simulink model "PV"  (Simulink 8.3)
settings: Solver=ode45  StartTime=0.0  StopTime=0.7  RelTol=1e-3
undefined symbols (not defined in the file or in its folder): ln
libraries: simulink x3, powerlib x1
settings Model: Creator=Birdman  LastModifiedBy=jt  SimulationMode=accelerator
settings OptimizationCC: InitFltsAndDblsToZero=on  EfficientMapNaN2IntZero=off
settings DebuggingCC: SaveWithParameterizedLinksMsg=none  SignalResolutionControl=TryResolveAllWithWarning  FcnCallInpInsideContextMsg=UseLocalSettings  StateNameClashWarn=none
settings HardwareCC: TargetIntDivRoundTo=Zero  TargetEndianess=LittleEndian  TargetHWDeviceType=MATLAB Host  ProdEqTarget=off
settings CodeAppCC: MaxIdLength=128
settings ConfigurationSet: Description=SimMechanics 2G

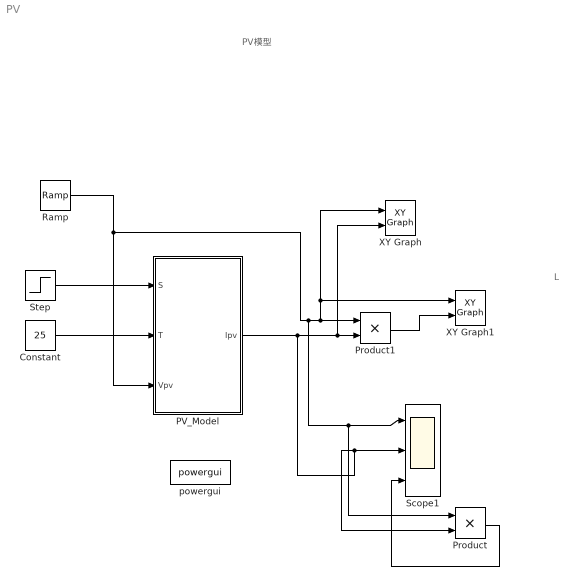
== system PV ==
  note: PV模型
  note: L
  Constant : Constant  Value=25
  PV_Model : Subsystem  mask{Vm=288, Im=13.88, Voc=354, Isc=14.88, Sref=1000, Tref=25, a=0.0025, b=0.0028, Rs=0.5}
      mask prompts: a "a(A/C)"; b "b(V/C)"
      mask Display: disp('PV_array')
  Product : Product
  Product1 : Product
  Ramp : simulink/Sources/Ramp  slope=800  start=0  X0=0
  Scope1 : Scope  NumInputPorts=3
      settings: YMin=255.75~14.58~3737.5  YMax=258.5~14.6125~3770
  Step : Step  Time=0.3  Before=1000  After=1000  SampleTime=0
  XY Graph : simulink/Sinks/XY Graph  xmin=0  xmax=400  ymin=0  ymax=20  st=-1
  XY Graph1 : simulink/Sinks/XY Graph  xmin=0  xmax=400  ymin=0  ymax=4100  st=-1
  powergui : powerlib/powergui  SimulationMode=Discrete  SolverType=Tustin  SampleTime=1e-6  frequency=60  SPID=off  DisableSnubberDevices=off  DisableRonSwitches=off  DisableVfSwitches=off  SwTol=0  Interpol=off  DisplayEquations=off  Ts=0  methode=off  frequencyindice=0  Pbase=100e6  ErrMax=1e-4  Iterations=50  UnitsV=kV  UnitsW=MW  FunctionMessages=off  echomessages=off  HookPort=off  EnableUseOfTLC=off  x0status=blocks  RestoreLinks=warning  ResistiveCurrentMeasurement=off  Frange=[0:2:500]  Ylog=off  Xlog=on  ShowGrid=off  save=off  variable=ZData  structure=io  ZoomFFT=off  StartTime=0.0  cycles=3  DisplayStyle=1  fundamental=50  FreqAxis=on  MaxFrequency=2500  frequencyindicesteady=1  RmsSteady=1  display=off
  wires:
  Step/1 -> PV_Model/1(S)
  Constant/1 -> PV_Model/2(T)
  Ramp/1 -> Product/1, Scope1/1, XY Graph/1, XY Graph1/1, Product1/1, PV_Model/3(Vpv)
  PV_Model/1(Ipv) -> Product/2, Scope1/2, XY Graph/2, Product1/2
  Product/1 -> Scope1/3
  Product1/1 -> XY Graph1/2

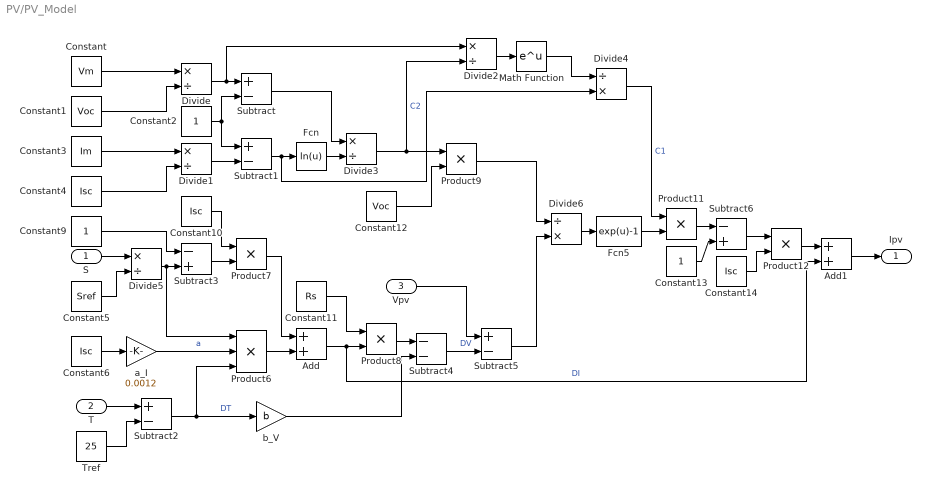
== system PV/PV_Model ==
  S : Inport
  T : Inport  Port=2
  Vpv : Inport  Port=3
  Add : Sum
  Add1 : Sum
  Constant : Constant  Value=Vm
  Constant1 : Constant  Value=Voc
  Constant{4,6,10,14} (4 alike) : Constant  Value=Isc
  Constant11 : Constant  Value=Rs
  Constant12 : Constant  Value=Voc
  Constant13 : Constant
  Constant2 : Constant
  Constant3 : Constant  Value=Im
  Constant5 : Constant  Value=Sref
  Constant9 : Constant
  Divide{,1..3,5} (5 alike) : Product  Inputs=*/
  Divide4 : Product  Inputs=/*
  Divide6 : Product  Inputs=/*
  Fcn : Fcn  Expr=ln(u)
  Fcn5 : Fcn  Expr=exp(u)-1
  Math Function : Math  SaturateOnIntegerOverflow=on
  Product{7..9,11..12} (5 alike) : Product  RndMeth=Zero
  Product6 : Product  Inputs=3  RndMeth=Zero
  Subtract{,1..2,5} (4 alike) : Sum  Inputs=+-
  Subtract3 : Sum  Inputs=-+
  Subtract4 : Sum  Inputs=--
  Subtract6 : Sum  Inputs=-+
  Tref : Constant  Value=25
  a_I : Gain  Gain=0.0012
  b_V : Gain  Gain=b
  Ipv : Outport
  wires:
  Constant1/1 -> Divide/2
  Constant/1 -> Divide/1
  Divide/1 -> Subtract/1, Divide2/1
  Constant2/1 -> Subtract/2, Subtract1/1
  Constant4/1 -> Divide1/2
  Constant3/1 -> Divide1/1
  Divide1/1 -> Subtract1/2
  Subtract1/1 -> Divide4/2, Fcn/1
  Subtract/1 -> Divide3/1
  Divide3/1 -> Product9/1, Divide2/2  "C2"
  Divide2/1 -> Math Function/1
  Math Function/1 -> Divide4/1
  Divide4/1 -> Product11/1  "C1"
  T/1 -> Subtract2/1
  Tref/1 -> Subtract2/2
  Subtract2/1 -> Product6/3, b_V/1  "DT"
  S/1 -> Divide5/1
  b_V/1 -> Subtract4/2
  Constant6/1 -> a_I/1
  a_I/1 -> Product6/2  "a"
  Divide5/1 -> Product6/1, Subtract3/2
  Constant9/1 -> Subtract3/1
  Subtract3/1 -> Product7/2
  Constant10/1 -> Product7/1
  Product7/1 -> Add/1
  Product6/1 -> Add/2
  Add/1 -> Product8/2, Add1/2  "DI"
  Constant11/1 -> Product8/1
  Product8/1 -> Subtract4/1
  Subtract4/1 -> Subtract5/2  "DV"
  Constant12/1 -> Product9/2
  Product9/1 -> Divide6/1
  Vpv/1 -> Subtract5/1
  Divide6/1 -> Fcn5/1
  Subtract5/1 -> Divide6/2
  Fcn5/1 -> Product11/2
  Product11/1 -> Subtract6/1
  Constant13/1 -> Subtract6/2
  Subtract6/1 -> Product12/1
  Constant14/1 -> Product12/2
  Product12/1 -> Add1/1
  Add1/1 -> Ipv/1
  Fcn/1 -> Divide3/2
  Constant5/1 -> Divide5/2
